simulink model "j01_McuInit"  (R2024a)
settings: Solver=FixedStepDiscrete  StartTime=0.0  StopTime=1  FixedStep=mSim.dTime  MaxStep=Define.sModelSampleTime  RelTol=7.1420e-05
undefined symbols (not defined in the file): CnstCnst, J01MINIT
settings Model: Creator=user  LastModifiedBy=admin
settings SolverCC: MaxConsecutiveZCs=10000  ZeroCrossAlgorithm=Adaptive  AlgebraicLoopSolver=TrustRegion
settings DataIOCC: SaveOutput=off  DSMLogging=off  InspectSignalLogs=on  SaveTime=off  SignalLoggingName=logsout_Validator
settings OptimizationCC: BlockReduction=off  DefaultParameterBehavior=Inlined  UseDivisionForNetSlopeComputation=UseDivisionForReciprocalsOfIntegersOnly  GainParamInheritBuiltInType=on  UseFloatMulNetSlope=on  DefaultUnderspecifiedDataType=single  InlineInvariantSignals=on  BitwiseOrLogicalOp=Logical operator  PassReuseOutputArgsAs=Individual arguments  EfficientFloat2IntCast=on  LifeSpan=Inf  OptimizeBlockOrder=speed  DifferentSizesBufferReuse=on  EfficientTunableParamExpr=on
settings DebuggingCC: SignalInfNanChecking=error  SignalRangeChecking=error  ReadBeforeWriteMsg=EnableAllAsError  WriteAfterWriteMsg=EnableAllAsError  WriteAfterReadMsg=EnableAllAsError  AlgebraicLoopMsg=error  ArtificialAlgebraicLoopMsg=error  SaveWithDisabledLinksMsg=error  SaveWithParameterizedLinksMsg=error  BlockPriorityViolationMsg=error  SolverPrmCheckMsg=error  InheritedTsInSrcMsg=error  SingleTaskRateTransMsg=error  TasksWithSamePriorityMsg=error  SigSpecEnsureSampleTimeMsg=error  CheckMatrixSingularityMsg=error  IntegerOverflowMsg=error  ParameterUnderflowMsg=error  ParameterPrecisionLossMsg=error  ParameterTunabilityLossMsg=error  UnderSpecifiedDataTypeMsg=error  UnnecessaryDatatypeConvMsg=warning  VectorMatrixConversionMsg=error  SignalLabelMismatchMsg=error  UnconnectedInputMsg=error  UnconnectedOutputMsg=error  UnconnectedLineMsg=error  SFcnCompatibilityMsg=error  UniqueDataStoreMsg=error  BusObjectLabelMismatch=error  RootOutportRequireBusObject=error  AssertControl=DisableAll  ModelReferenceIOMismatchMessage=error  UnknownTsInhSupMsg=error  ModelReferenceDataLoggingMessage=error  ModelReferenceSymbolNameMessage=none  StateNameClashWarn=warning  StrictBusMsg=ErrorOnBusTreatedAsVector  NonBusSignalsTreatedAsBus=error  SFInvalidInputDataAccessInChartInitDiag=error  SFTransitionOutsideNaturalParentDiag=error  SFUnreachableExecutionPathDiag=error  SFUndirectedBroadcastEventsDiag=error  SFTransitionActionBeforeConditionDiag=error  SFTemporalDelaySmallerThanSampleTimeDiag=error  SFSelfTransitionDiag=error  SFExecutionAtInitializationDiag=error  IntegerSaturationMsg=error  UnitsInconsistencyMsg=none  VariantConditionMismatch=error
settings HardwareCC: ProdBitPerChar=16  ProdBitPerInt=16  ProdBitPerPointer=32  ProdBitPerSizeT=32  ProdBitPerPtrDiffT=32  ProdLargestAtomicInteger=Integer  ProdLargestAtomicFloat=None  ProdWordSize=16  ProdLongLongMode=on  ProdHWDeviceType=Texas Instruments->C2000
settings ModelReferenceCC: EnableRefExpFcnMdlSchedulingChecks=on  ModelReferenceNumInstancesAllowed=Single
settings SFSimCC: SimUseLocalCustomCode=off  CompileTimeRecursionLimit=0  EnableRuntimeRecursion=off  MATLABDynamicMemAlloc=off  CustomCodeUndefinedFunction=UseInterfaceOnly
settings RTWCC: Description=Embedded Coder  SystemTargetFile=ert.tlc  GenCodeOnly=on  TemplateMakefile=ert_default_tmf  GenerateReport=on  RTWUseLocalCustomCode=off  BuildConfiguration=Faster Runs  IncludeHyperlinkInReport=on  LaunchReport=on  GenerateTraceInfo=on  GenerateTraceReport=on  GenerateTraceReportSl=on  GenerateTraceReportSf=on  GenerateWebview=on  GenerateCodeMetricsReport=on  GenerateCodeReplacementReport=on  GPUComputeCapability=3.5  DLArmComputeVersion=19.05
settings CodeAppCC: ForceParamTrailComments=on  IgnoreCustomStorageClasses=off  MATLABFcnDesc=on  MangleLength=4  CustomSymbolStrGlobalVar=GvJ01$N$M  CustomSymbolStrType=StrJ01$N$M  CustomSymbolStrFcn=$N$M$F  CustomSymbolStrMacro=$N$M  DefineNamingRule=UpperCase  ParamNamingRule=UpperCase  SimulinkBlockComments=off  MATLABSourceComments=on  EnableCustomComments=on  ReqsInCode=on
settings ERTTargetCC: TargetLangStandard=C99 (ISO)  UtilityFuncGeneration=Shared location  MultiwordLength=2048  IncludeMdlTerminateFcn=off  CombineSignalStateStructs=on  SuppressErrorStatus=on  SupportAbsoluteTime=off  SupportNonFinite=off  ParenthesesLevel=Maximum  CastingMode=Standards  GenerateSharedConstants=off  InlinedParameterPlacement=NonHierarchical  ERTSrcFileBannerTemplate=t_code_template.cgt  ERTHdrFileBannerTemplate=t_code_template.cgt  ERTDataSrcFileTemplate=t_code_template.cgt  ERTDataHdrFileTemplate=t_code_template.cgt  ERTCustomFileTemplate=example_file_process.tlc  ERTFilePackagingFormat=CompactWithDataFile  PreserveExpressionOrder=on  SuppressUnreachableDefaultCases=off  EnableSignedLeftShifts=off  EnableSignedRightShifts=off  IndentStyle=Allman  IndentSize=4
settings ConfigComp: CovSaveName=coveragedata  CovMetricSettings=we  CovEnableCumulative=off  CovSaveCumulativeToWorkspaceVar=on  CovSaveSingleToWorkspaceVar=on  CovOutputDir=sldv_output/$ModelName$\sldv_covoutput  PSVerificationMode=BugFinder  PSModelRefIgnoreList=[]  PSEnableModelRefIgnoreList=off  PSModelRefMinMaxVerif=CheckAndConstrain  PSAutoStubLUT=on  DVModelCoverageObjectives=MCDC  DVTestSuiteOptimization=CombinedObjectives (Nonlinear Extended)  DVRebuildModelRepresentation=Always
settings SimscapeCC: SimscapeNormalizeSystem=off

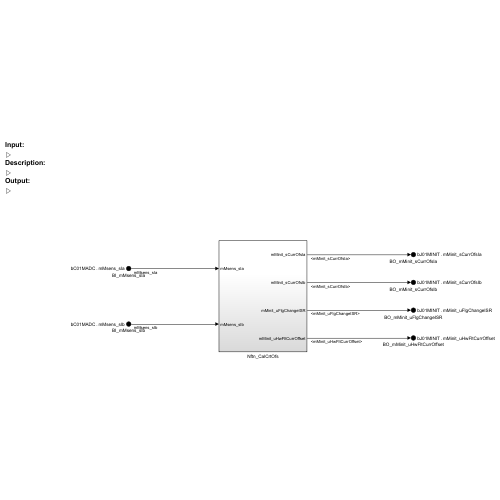
[thumbnail: Simulink's stored preview of the top-level diagram]
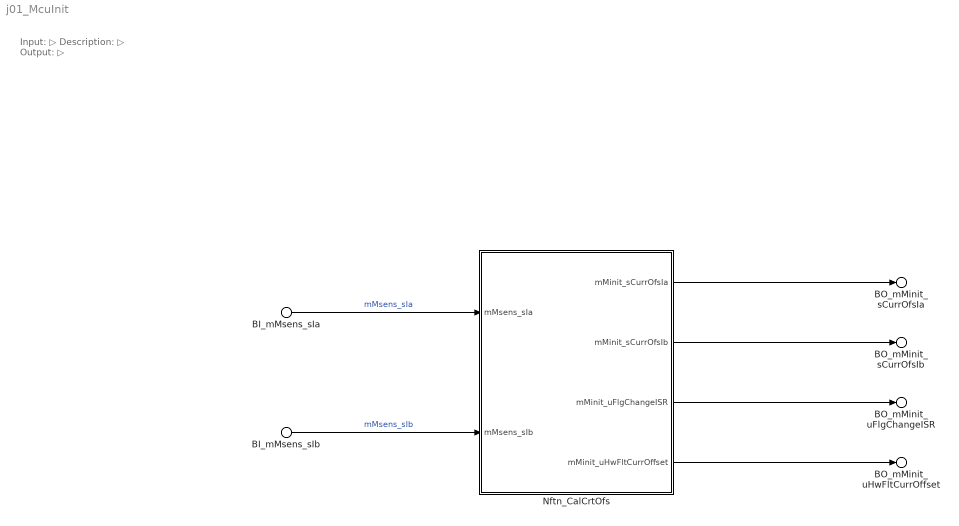
== system j01_McuInit ==
  note: Input:
      | ▷
      | Description:
      | ▷
      | Output:
      | ▷
  BI_mMsens_sIa : Inport  Description=■ 설명: A상 전류  PortName=bC01MADC  Element=mMsens_sIa
  BI_mMsens_sIb : Inport  Description=■ 설명: B상 전류  PortName=bC01MADC  Element=mMsens_sIb
  Nftn_CalCrtOfs : Subsystem
      settings: RTWSystemCode=Nonreusable function  RTWFcnNameOpts=Use subsystem name
  BO_mMinit_sCurrOfsIa : Outport  Description=■ 설명: A상 전류 센서 오프셋  PortName=bJ01MINIT  Element=mMinit_sCurrOfsIa
  BO_mMinit_sCurrOfsIb : Outport  Description=■ 설명: B상 전류 센서 오프셋  PortName=bJ01MINIT  Element=mMinit_sCurrOfsIb
  BO_mMinit_uFlgChangeISR : Outport  Description=■ 설명: 인터럽트 변경 Flag  PortName=bJ01MINIT  Element=mMinit_uFlgChangeISR
  BO_mMinit_uHwFltCurrOffset : Outport  Description=■ 설명: 전류 센서 오프셋 고장 신호  PortName=bJ01MINIT  Element=mMinit_uHwFltCurrOffset
  wires:
  Nftn_CalCrtOfs/1(mMinit_sCurrOfsIa) -> BO_mMinit_sCurrOfsIa/1
  BI_mMsens_sIb/1 -> Nftn_CalCrtOfs/2(mMsens_sIb)  "mMsens_sIb"
  Nftn_CalCrtOfs/3(mMinit_uFlgChangeISR) -> BO_mMinit_uFlgChangeISR/1
  Nftn_CalCrtOfs/2(mMinit_sCurrOfsIb) -> BO_mMinit_sCurrOfsIb/1
  BI_mMsens_sIa/1 -> Nftn_CalCrtOfs/1(mMsens_sIa)  "mMsens_sIa"
  Nftn_CalCrtOfs/4(mMinit_uHwFltCurrOffset) -> BO_mMinit_uHwFltCurrOffset/1

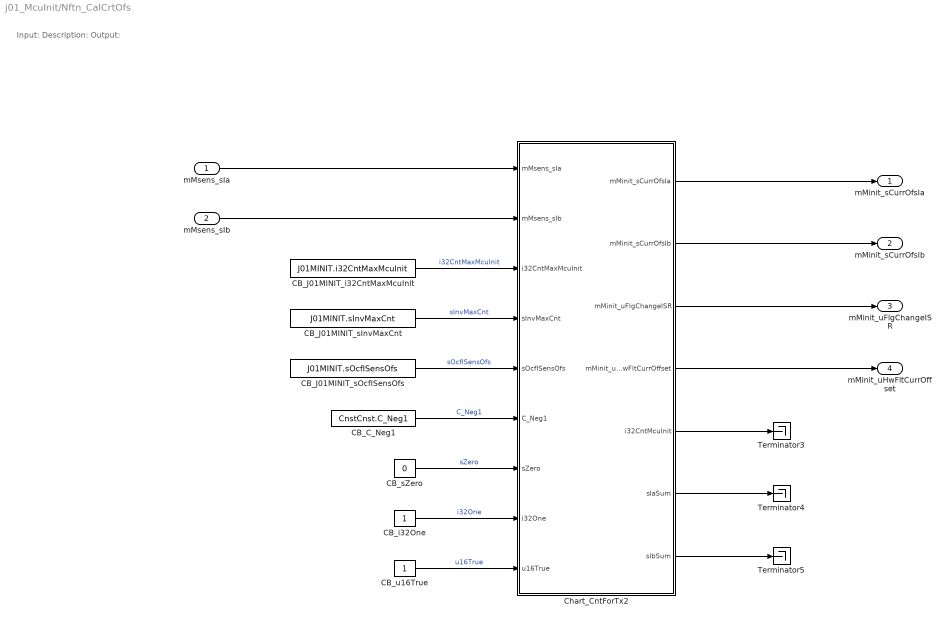
== system j01_McuInit/Nftn_CalCrtOfs ==
  note: Input:
      | Description:
      | Output:
  mMsens_sIa : Inport  Description=■ 설명: 모터 A상 전류  OutMin=-162.6  OutMax=162.6
  mMsens_sIb : Inport  Description=■ 설명: 모터 B상 전류  Port=2  OutMin=-162.6  OutMax=162.6
  CB_C_Neg1 : Constant  Value=CnstCnst.C_Neg1
  CB_J01MINIT_i32CntMaxMcuInit : Constant  Value=J01MINIT.i32CntMaxMcuInit
  CB_J01MINIT_sInvMaxCnt : Constant  Value=J01MINIT.sInvMaxCnt
  CB_J01MINIT_sOcfISensOfs : Constant  Value=J01MINIT.sOcfISensOfs
  CB_i32One : Constant  OutDataTypeStr=int32
  CB_sZero : Constant  Value=0  OutDataTypeStr=single
  CB_u16True : Constant  OutDataTypeStr=uint16
  Chart_CntForTx2 : Stateflow chart  TreatAsAtomicUnit=on
  Terminator3 : Terminator
  Terminator4 : Terminator
  Terminator5 : Terminator
  mMinit_sCurrOfsIa : Outport  Description=■ 설명: A상 Offset 전류  OutMin=-162.6  OutMax=162.6
  mMinit_sCurrOfsIb : Outport  Description=■ 설명: B상 Offset 전류  Port=2  OutMin=-162.6  OutMax=162.6
  mMinit_uFlgChangeISR : Outport  Description=■ 설명: 인터럽트 활성화 신호  Port=3  OutMin=0  OutMax=1
  mMinit_uHwFltCurrOffset : Outport  Description="■ 설명: Current  Sensors Offset Error"  Port=4  OutMin=0  OutMax=1
  wires:
  CB_i32One/1 -> Chart_CntForTx2/8(i32One)  "i32One"
  CB_J01MINIT_i32CntMaxMcuInit/1 -> Chart_CntForTx2/3(i32CntMaxMcuInit)  "i32CntMaxMcuInit"
  mMsens_sIb/1 -> Chart_CntForTx2/2(mMsens_sIb)
  mMsens_sIa/1 -> Chart_CntForTx2/1(mMsens_sIa)
  CB_J01MINIT_sInvMaxCnt/1 -> Chart_CntForTx2/4(sInvMaxCnt)  "sInvMaxCnt"
  CB_sZero/1 -> Chart_CntForTx2/7(sZero)  "sZero"
  Chart_CntForTx2/2(mMinit_sCurrOfsIb) -> mMinit_sCurrOfsIb/1
  Chart_CntForTx2/1(mMinit_sCurrOfsIa) -> mMinit_sCurrOfsIa/1
  CB_C_Neg1/1 -> Chart_CntForTx2/6(C_Neg1)  "C_Neg1"
  CB_J01MINIT_sOcfISensOfs/1 -> Chart_CntForTx2/5(sOcfISensOfs)  "sOcfISensOfs"
  CB_u16True/1 -> Chart_CntForTx2/9(u16True)  "u16True"
  Chart_CntForTx2/3(mMinit_uFlgChangeISR) -> mMinit_uFlgChangeISR/1
  Chart_CntForTx2/4(mMinit_uHwFltCurrOffset) -> mMinit_uHwFltCurrOffset/1
  Chart_CntForTx2/5(i32CntMcuInit) -> Terminator3/1
  Chart_CntForTx2/6(sIaSum) -> Terminator4/1
  Chart_CntForTx2/7(sIbSum) -> Terminator5/1

== stateflow chart j01_McuInit/Nftn_CalCrtOfs/Chart_CntForTx2 ==
  (default) -> (junction 2)
  (junction 2) -> (junction 3) [order 1] : [i32CntMcuInit >= i32CntMaxMcuInit]
  (junction 2) -> (junction 13) [order 2] : {
      | i32CntMcuInit = i32CntMcuInit + i32One;
      | sIaSum += mMsens_sIa;
      | sIbSum += mMsens_sIb;
      | }
  (junction 3) -> (junction 80) : {
      | i32CntMcuInit = i32CntMaxMcuInit;
      | mMinit_sCurrOfsIa = sIaSum * sInvMaxCnt;
      | mMinit_sCurrOfsIb = sIbSum * sInvMaxCnt;
      | }
  (junction 80) -> (junction 81) [order 1] : [mMinit_sCurrOfsIa < sZero]
  (junction 80) -> (junction 82) [order 2] : {
      | sLocalCurrOfsIa = mMinit_sCurrOfsIa;
      | }
  (junction 81) -> (junction 83) : {
      | sLocalCurrOfsIa = mMinit_sCurrOfsIa * C_Neg1;
      | }
  (junction 83) -> (junction 82)
  (junction 82) -> (junction 98)
  (junction 98) -> (junction 101) [order 1] : [mMinit_sCurrOfsIb < sZero]
  (junction 98) -> (junction 104) [order 2] : {
      | sLocalCurrOfsIb = mMinit_sCurrOfsIb;
      | }
  (junction 101) -> (junction 105) : {
      | sLocalCurrOfsIb = mMinit_sCurrOfsIb * C_Neg1;
      | }
  (junction 105) -> (junction 104)
  (junction 104) -> (junction 120)
  (junction 120) -> (junction 127) [order 1] : [(sLocalCurrOfsIa > sOcfISensOfs)||(sLocalCurrOfsIb > sOcfISensOfs)]
  (junction 120) -> (junction 124) [order 2] : /* No Action */
  (junction 127) -> (junction 122) : {
      | mMinit_uHwFltCurrOffset = u16True;
      | }
  (junction 122) -> (junction 124)
  (junction 124) -> (junction 4) : {
      | mMinit_uFlgChangeISR = u16True;
      | }
  (junction 4) -> (junction 13)
  (junction 13) -> (junction 34)
  data: mMinit_sCurrOfsIa output single; mMinit_sCurrOfsIb output single; mMinit_uFlgChangeISR output uint16; mMinit_uHwFltCurrOffset output uint16; mMsens_sIa input; mMsens_sIb input; i32CntMcuInit output int32 =1; i32CntMaxMcuInit input int32; sInvMaxCnt input; sOcfISensOfs input; C_Neg1 input; sZero input; i32One input; sIaSum output single; sIbSum output single; sLocalCurrOfsIa local single; sLocalCurrOfsIb local single; u16True input
